simulink model "model"  (R2016a)
settings: Solver=VariableStepAuto  StartTime=0.0  StopTime=Data(end,1)  FixedStep=1  MaxStep=1  RelTol=1e-3
values from neighbouring files (symbols this model uses):
  Data = [0 60 120 180 240 300 360 420 480 540 600 660 ... (858 elements, 286x3)]    [DataBoiler.mat]
  lambda = 78    [createW.m]
libraries: simulink x2, cstblocks x1
settings Model: Creator=ivand  LastModifiedBy=ivand

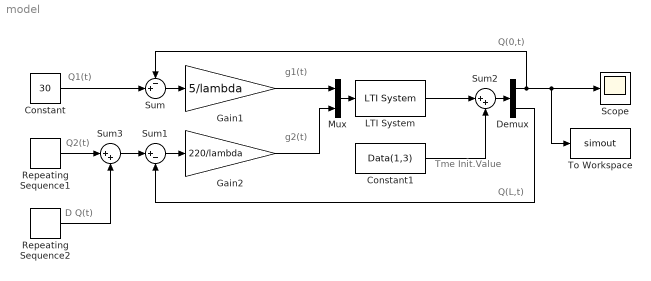
== system model ==
  note: Tme Init.Value
  note: g1(t)
  note: D Q(t)
  note: Q2(t)
  note: Q1(t)
  note: g2(t)
  note: Q(0,t)
  note: Q(L,t)
  Constant : Constant  Value=30
  Constant1 : Constant  Value=Data(1,3)
  Demux : Demux  Outputs=2
  Gain1 : Gain  Gain=5/lambda
  Gain2 : Gain  Gain=220/lambda
  LTI System : cstblocks/LTI System  sys=W  IC=[]
  Mux : Mux  Inputs=2
  Repeating Sequence1 : simulink/Sources/Repeating Sequence  rep_seq_t=Data(:,1)  rep_seq_y=Data(:,2)
  Repeating Sequence2 : simulink/Sources/Repeating Sequence  rep_seq_t=tu  rep_seq_y=u
  Scope : Scope
  Sum : Sum  Inputs=-+|
  Sum1 : Sum  Inputs=|+-
  Sum2 : Sum  Inputs=|++
  Sum3 : Sum  Inputs=|++
  To Workspace : ToWorkspace  VariableName=simout  SampleTime=-1
  wires:
  Constant/1 -> Sum/2
  Sum3/1 -> Sum1/1
  Demux/2 -> Sum1/2
  Sum/1 -> Gain1/1
  Sum1/1 -> Gain2/1
  Gain1/1 -> Mux/1
  Gain2/1 -> Mux/2
  Mux/1 -> LTI System/1
  Repeating Sequence1/1 -> Sum3/1
  Repeating Sequence2/1 -> Sum3/2
  Demux/1 -> Scope/1, To Workspace/1, Sum/1
  Sum2/1 -> Demux/1
  LTI System/1 -> Sum2/1
  Constant1/1 -> Sum2/2
